simulink model "lotka_volterra"  (R2023b)
settings: Solver=VariableStepAuto  StartTime=0.0  StopTime=25  RelTol=1e-3
settings Model: Creator=Nishanth S  LastModifiedBy=Nishanth S

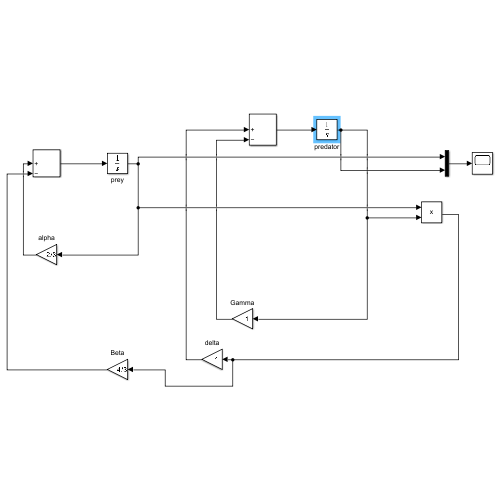
[thumbnail: Simulink's stored preview of the top-level diagram]
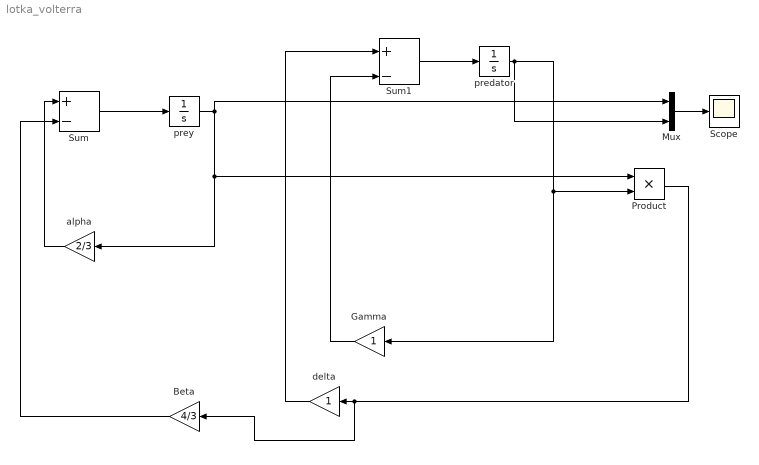
== system lotka_volterra ==
  Beta : Gain  Gain=4/3
  Gamma : Gain
  Mux : Mux  Inputs=2
  Product : Product
  Scope : Scope
  Sum : Sum  Inputs=|+-
  Sum1 : Sum  Inputs=|+-
  alpha : Gain  Gain=2/3
  delta : Gain
  predator : Integrator  InitialCondition=1.5
  prey : Integrator  InitialCondition=1.2
  wires:
  Sum/1 -> prey/1
  prey/1 -> Mux/1, Product/1, alpha/1
  alpha/1 -> Sum/1
  Sum1/1 -> predator/1
  predator/1 -> Mux/2, Product/2, Gamma/1
  Gamma/1 -> Sum1/2
  Product/1 -> Beta/1, delta/1
  delta/1 -> Sum1/1
  Beta/1 -> Sum/2
  Mux/1 -> Scope/1
